simulink model "gate_gearbox_pid"  (R2025b)
settings: Solver=ode4  StartTime=0.0  StopTime=8  FixedStep=0.001  RelTol=1e-3
settings Model: Creator=Majesty  LastModifiedBy=Majesty

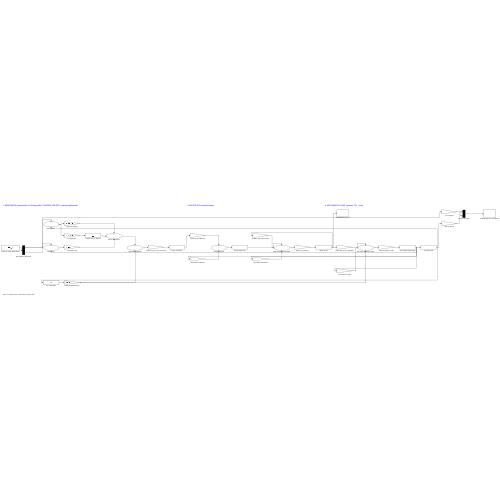
[thumbnail: Simulink's stored preview of the top-level diagram]
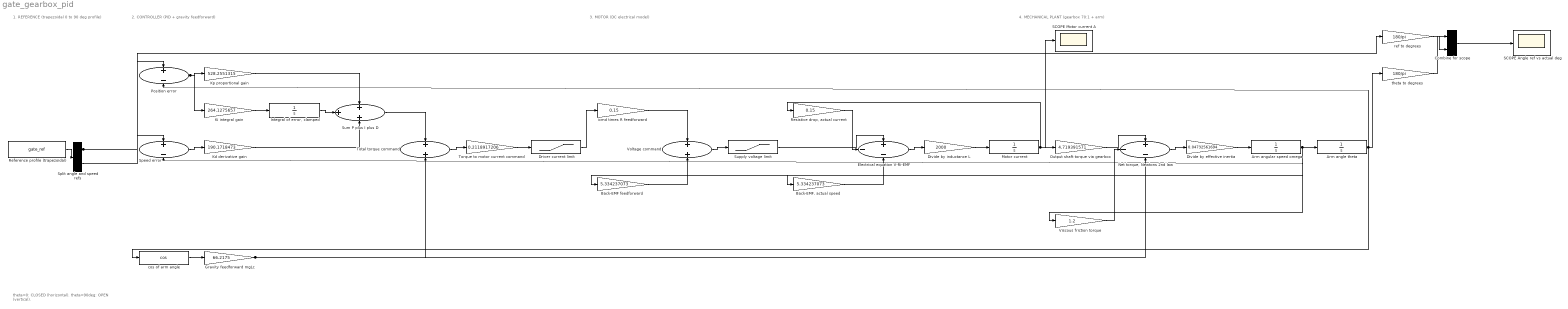
== system gate_gearbox_pid ==
  note: 1. REFERENCE (trapezoidal 0 to 90 deg profile)
  note: 2. CONTROLLER (PID + gravity feedforward)
  note: 3. MOTOR (DC electrical model)
  note: 4. MECHANICAL PLANT (gearbox 70:1 + arm)
  note: theta=0: CLOSED (horizontal). theta=90deg: OPEN (vertical).
  Arm angle theta : Integrator
  Arm angular speed omega : Integrator
  Back-EMF feedforward : Gain  Gain=5.334237073
  "Back-EMF, actual speed" : Gain  Gain=5.334237073
  Combine for scope : Mux  Inputs=2
  Divide by effective inertia : Gain  Gain=0.04732561694
  Divide by inductance L : Gain  Gain=2000
  Driver current limit : Saturate  UpperLimit=30  LowerLimit=-30
  Electrical equation V-Ri-EMF : Sum  Inputs=+--
  Gravity feedforward mgLc : Gain  Gain=66.2175
  "Integral of error, clamped" : Integrator  LimitOutput=on  UpperSaturationLimit=300  LowerSaturationLimit=-300
  Kd derivative gain : Gain  Gain=190.1718473
  Ki integral gain : Gain  Gain=264.1275657
  Kp proportional gain : Gain  Gain=528.2551315
  Motor current : Integrator
  "Net torque, Newtons 2nd law" : Sum  Inputs=+--
  Output shaft torque via gearbox : Gain  Gain=4.719391571
  Position error : Sum  Inputs=+-
  Reference profile (trapezoidal) : FromWorkspace  VariableName=gate_ref
  "Resistive drop, actual current" : Gain  Gain=0.15
  SCOPE Angle ref vs actual deg : Scope
  SCOPE Motor current A : Scope
  Speed error : Sum  Inputs=+-
  Split angle and speed refs : Demux  Outputs=2
  Sum P plus I plus D : Sum  Inputs=+++
  Supply voltage limit : Saturate  UpperLimit=24  LowerLimit=-24
  Torque to motor current command : Gain  Gain=0.2118917206
  Total torque command : Sum
  Viscous friction torque : Gain  Gain=1.2
  Voltage command : Sum
  cos of arm angle : Trigonometry  Operator=cos
  icmd times R feedforward : Gain  Gain=0.15
  ref to degrees : Gain  Gain=180/pi
  theta to degrees : Gain  Gain=180/pi
  wires:
  Reference profile (trapezoidal)/1 -> Split angle and speed refs/1
  Split angle and speed refs/1 -> Position error/1, ref to degrees/1
  Split angle and speed refs/2 -> Speed error/1
  Arm angle theta/1 -> Position error/2, cos of arm angle/1, theta to degrees/1
  Arm angular speed omega/1 -> Speed error/2, Back-EMF feedforward/1, "Back-EMF, actual speed"/1, Viscous friction torque/1, Arm angle theta/1
  cos of arm angle/1 -> Gravity feedforward mgLc/1
  Gravity feedforward mgLc/1 -> Total torque command/2, "Net torque, Newtons 2nd law"/3
  Position error/1 -> Kp proportional gain/1, Ki integral gain/1
  Kp proportional gain/1 -> Sum P plus I plus D/1
  Ki integral gain/1 -> "Integral of error, clamped"/1
  "Integral of error, clamped"/1 -> Sum P plus I plus D/2
  Speed error/1 -> Kd derivative gain/1
  Kd derivative gain/1 -> Sum P plus I plus D/3
  Sum P plus I plus D/1 -> Total torque command/1
  Total torque command/1 -> Torque to motor current command/1
  Torque to motor current command/1 -> Driver current limit/1
  Driver current limit/1 -> icmd times R feedforward/1
  Back-EMF feedforward/1 -> Voltage command/2
  icmd times R feedforward/1 -> Voltage command/1
  Voltage command/1 -> Supply voltage limit/1
  Supply voltage limit/1 -> Electrical equation V-Ri-EMF/1
  "Resistive drop, actual current"/1 -> Electrical equation V-Ri-EMF/2
  "Back-EMF, actual speed"/1 -> Electrical equation V-Ri-EMF/3
  Electrical equation V-Ri-EMF/1 -> Divide by inductance L/1
  Divide by inductance L/1 -> Motor current/1
  Motor current/1 -> "Resistive drop, actual current"/1, Output shaft torque via gearbox/1, SCOPE Motor current A/1
  Output shaft torque via gearbox/1 -> "Net torque, Newtons 2nd law"/1
  Viscous friction torque/1 -> "Net torque, Newtons 2nd law"/2
  "Net torque, Newtons 2nd law"/1 -> Divide by effective inertia/1
  Divide by effective inertia/1 -> Arm angular speed omega/1
  theta to degrees/1 -> Combine for scope/1
  ref to degrees/1 -> Combine for scope/2
  Combine for scope/1 -> SCOPE Angle ref vs actual deg/1
